simulink library "Gain_and_Thresh"  (R2023a)
settings: Solver=VariableStepAuto  StartTime=0.0  StopTime=10.0  RelTol=1e-3
settings Model: Creator=ADMIN  LastModifiedBy=ADMIN

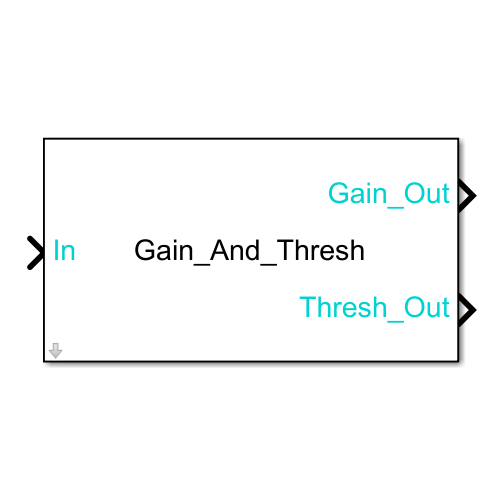
[thumbnail: Simulink's stored preview of the top-level diagram]
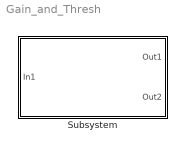
== system Gain_and_Thresh ==
  Subsystem : Subsystem  mask{GAIN=0, CONSTANT=0}
      mask Display:
      | disp('Gain_And_Thresh')
      | color('cyan');
      | port_label('input', 1, 'In');
      | port_label('output', 1, 'Gain_Out');
      | port_label('output', 2, 'Thresh_Out');

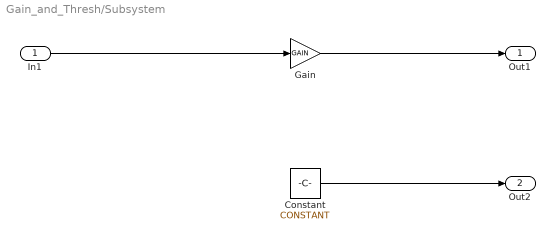
== system Gain_and_Thresh/Subsystem ==
  In1 : Inport
  Constant : Constant  Value=CONSTANT
  Gain : Gain  Gain=GAIN
  Out1 : Outport
  Out2 : Outport  Port=2
  wires:
  Gain/1 -> Out1/1
  Constant/1 -> Out2/1
  In1/1 -> Gain/1
